simulink model "dyn_ext_simple_test"  (R2015b)
settings: Solver=VariableStepAuto  StartTime=0.0  StopTime=4  FixedStep=0.001  RelTol=1e-3
settings Model: ExtModeTrigDuration=5000  Creator=robertph  LastModifiedBy=robertph
settings SolverCC: ZeroCrossControl=DisableAll  PositivePriorityOrder=on
settings RTWCC: SystemTargetFile=quarc_win64.tlc  TemplateMakefile=quarc_default_tmf  Description=QUARC Win64 Target
settings STFCustomTargetCC: GeneratePreprocessorConditionals=Use local settings  CPPClassGenCompliant=off
settings GRTTargetCC: ParMdlRefBuildCompliant=off  CompOptLevelCompliant=off  CombineOutputUpdateFcns=off  MatFileLogging=off  CPPClassGenCompliant=off  GRTInterface=on  UseToolchainInfoCompliant=off  ExtMode=on  ExtModeMexFile=quarc_comm

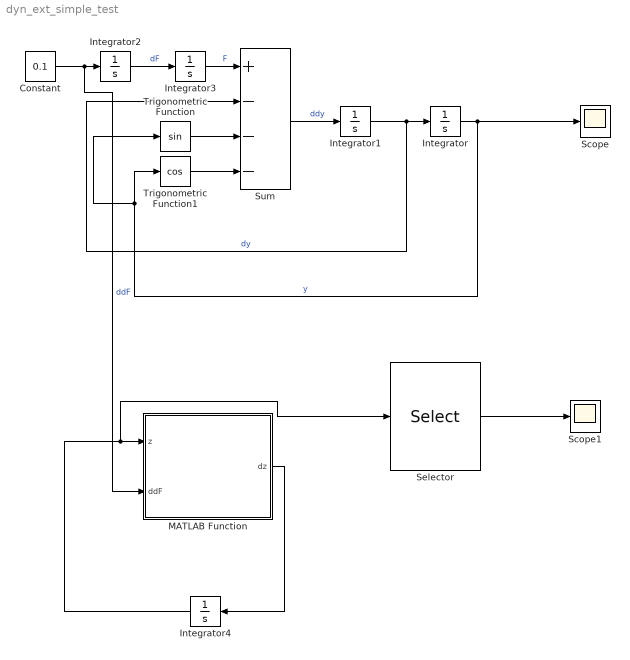
== system dyn_ext_simple_test ==
  Constant : Constant  Value=0.1
  Integrator{,1..3} (4 alike) : Integrator
  Integrator4 : Integrator  InitialCondition=[0; 0; -1; 1]
  MATLAB Function : MATLAB Function  TreatAsAtomicUnit=on
  Scope : Scope
  Scope1 : Scope
  Selector : Selector  InputPortWidth=4  IndexOptions=Index vector (dialog)  Indices=[1]  OutputSizes=1
  Sum : Sum  Inputs=+---
  Trigonometric Function : Trigonometry
  Trigonometric Function1 : Trigonometry  Operator=cos
  wires:
  Integrator1/1 -> Sum/2, Integrator/1  "dy"
  Sum/1 -> Integrator1/1  "ddy"
  Trigonometric Function/1 -> Sum/3
  Trigonometric Function1/1 -> Sum/4
  Integrator/1 -> Scope/1, Trigonometric Function1/1, Trigonometric Function/1  "y"
  Integrator2/1 -> Integrator3/1  "dF"
  Integrator3/1 -> Sum/1  "F"
  Constant/1 -> MATLAB Function/2(ddF), Integrator2/1  "ddF"
  MATLAB Function/1(dz) -> Integrator4/1
  Integrator4/1 -> Selector/1, MATLAB Function/1(z)
  Selector/1 -> Scope1/1

== matlab function dyn_ext_simple_test/MATLAB Function ==
  data: z input; dz output; ddF input
function dz = fcn(z, ddF)
%#codegen
%% x = phi^-1 (z)
x1 = z(1);
x2 = z(2);
x3 = z(3) + z(2) + sin(z(1)) + cos(z(1));
x4 = z(4) - z(2) - (1+z(2))*sin(z(1)) - (1 - z(2)) * cos(z(1));

%% alpha(x) and beta(x)
alpha = x2*(x2*(sin(x1)+cos(x1))-sin(x1)+cos(x1))-x4+(sin(x1)-cos(x1)+1)*(-x2+x3-sin(x1)-cos(x1));
beta = 1;

%% dz
dz = zeros(4, 1);
dz(1) = z(2);
dz(2) = z(3);
dz(3) = z(4);
dz(4) = alpha + beta * ddF;
